simulink library "CTRL_SPECCTRL"  (R2024b)
settings: Solver=VariableStepAuto  StartTime=0.0  StopTime=10.0  RelTol=1e-3
libraries: CTRL_SPECCTRL_COND x1, CTRL_SPECCTRL_FB x1, CTRL_SPECCTRL_FF x1
settings Model: Creator=blatak  LastModifiedBy=blatak

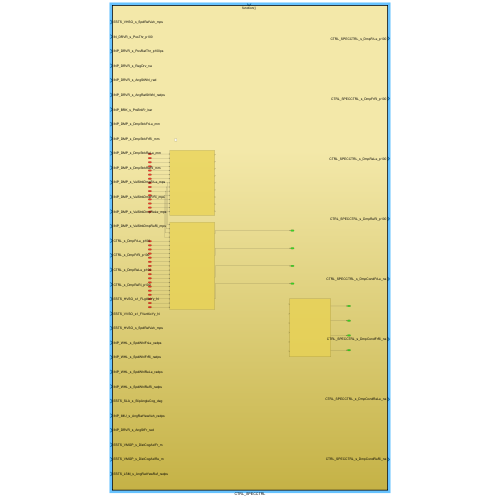
[thumbnail: Simulink's stored preview of the top-level diagram]
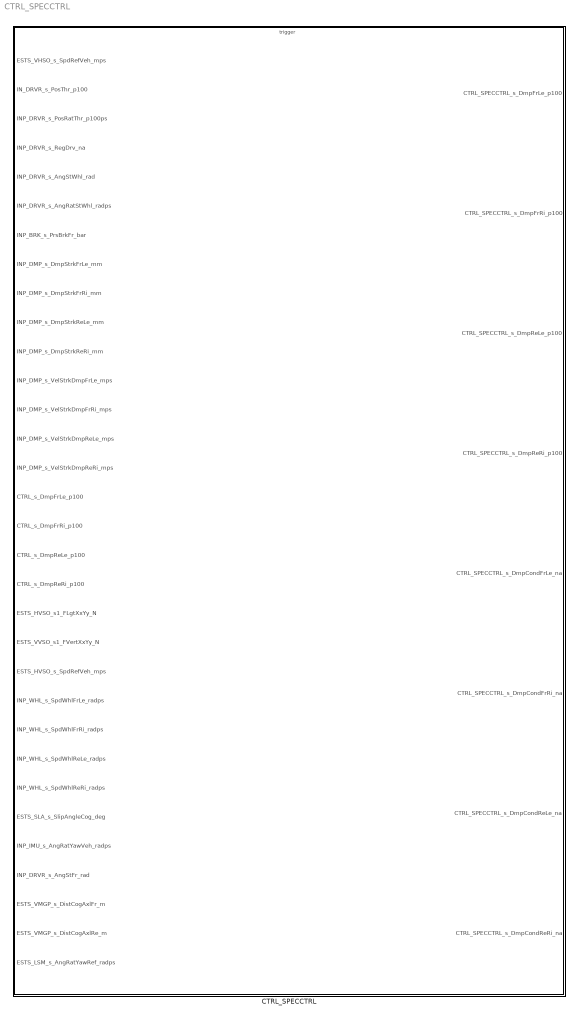
== system CTRL_SPECCTRL ==
  CTRL_SPECCTRL : Subsystem  TreatAsAtomicUnit=on

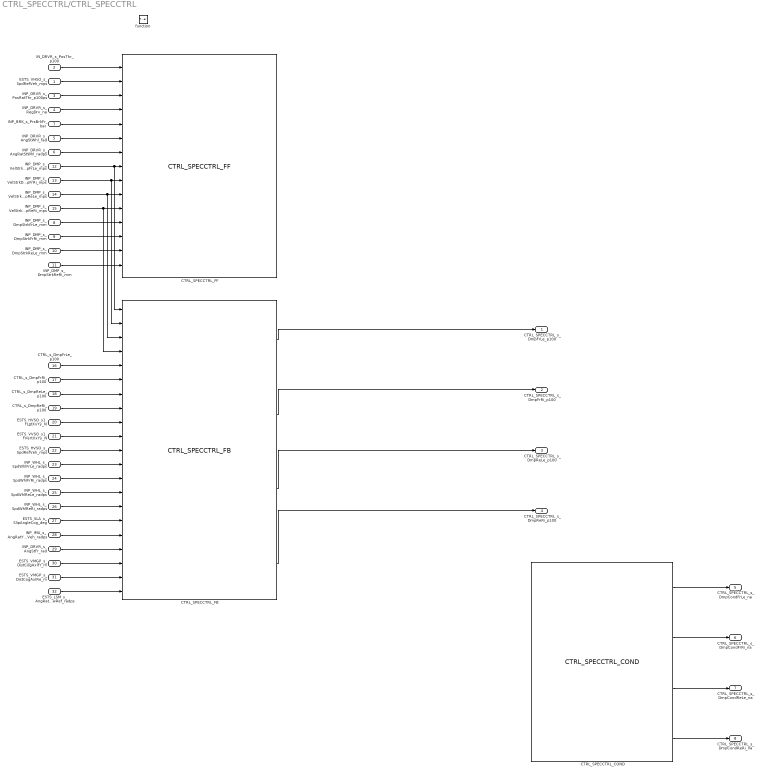
== system CTRL_SPECCTRL/CTRL_SPECCTRL ==
  ESTS_VHSO_s_SpdRefVeh_mps : Inport
  IN_DRVR_s_PosThr_p100 : Inport  Port=2
  INP_DRVR_s_PosRatThr_p100ps : Inport  Port=3
  INP_DRVR_s_RegDrv_na : Inport  Port=4
  INP_DRVR_s_AngStWhl_rad : Inport  Port=5
  INP_DRVR_s_AngRatStWhl_radps : Inport  Port=6
  INP_BRK_s_PrsBrkFr_bar : Inport  Port=7
  INP_DMP_s_DmpStrkFrLe_mm : Inport  Port=8
  INP_DMP_s_DmpStrkFrRi_mm : Inport  Port=9
  INP_DMP_s_DmpStrkReLe_mm : Inport  Port=10
  INP_DMP_s_DmpStrkReRi_mm : Inport  Port=11
  INP_DMP_s_VelStrkDmpFrLe_mps : Inport  Port=12
  INP_DMP_s_VelStrkDmpFrRi_mps : Inport  Port=13
  INP_DMP_s_VelStrkDmpReLe_mps : Inport  Port=14
  INP_DMP_s_VelStrkDmpReRi_mps : Inport  Port=15
  CTRL_s_DmpFrLe_p100 : Inport  Port=16
  CTRL_s_DmpFrRi_p100 : Inport  Port=17
  CTRL_s_DmpReLe_p100 : Inport  Port=18
  CTRL_s_DmpReRi_p100 : Inport  Port=19
  ESTS_HVSO_s1_FLgtXxYy_N : Inport  Port=20
  ESTS_VVSO_s1_FVertXxYy_N : Inport  Port=21
  ESTS_HVSO_s_SpdRefVeh_mps : Inport  Port=22
  INP_WHL_s_SpdWhlFrLe_radps : Inport  Port=23
  INP_WHL_s_SpdWhlFrRi_radps : Inport  Port=24
  INP_WHL_s_SpdWhlReLe_radps : Inport  Port=25
  INP_WHL_s_SpdWhlReRi_radps : Inport  Port=26
  ESTS_SLA_s_SlipAngleCog_deg : Inport  Port=27
  INP_IMU_s_AngRatYawVeh_radps : Inport  Port=28
  INP_DRVR_s_AngStFr_rad : Inport  Port=29
  ESTS_VMGP_s_DistCogAxlFr_m : Inport  Port=30
  ESTS_VMGP_s_DistCogAxlRe_m : Inport  Port=31
  ESTS_LSM_s_AngRatYawRef_radps : Inport  Port=32
  function : TriggerPort  TriggerType=function-call  VariantControl=(inherit)
  CTRL_SPECCTRL_COND : CTRL_SPECCTRL_COND/CTRL_SPECCTRL_COND  SystemSampleTime=-1  VariantActivationTime=update diagram  AllowFlexibleInterface=on  Latency=0  AutoFrameSizeCalculation=off
  CTRL_SPECCTRL_FB : CTRL_SPECCTRL_FB/CTRL_SPECCTRL_FB  SystemSampleTime=-1  VariantActivationTime=update diagram  AllowFlexibleInterface=on  Latency=0  AutoFrameSizeCalculation=off
  CTRL_SPECCTRL_FF : CTRL_SPECCTRL_FF/CTRL_SPECCTRL_FF  SystemSampleTime=-1  VariantActivationTime=update diagram  AllowFlexibleInterface=on  Latency=0  AutoFrameSizeCalculation=off
  CTRL_SPECCTRL_s_DmpFrLe_p100 : Outport
  CTRL_SPECCTRL_s_DmpFrRi_p100 : Outport  Port=2
  CTRL_SPECCTRL_s_DmpReLe_p100 : Outport  Port=3
  CTRL_SPECCTRL_s_DmpReRi_p100 : Outport  Port=4
  CTRL_SPECCTRL_s_DmpCondFrLe_na : Outport  Port=5
  CTRL_SPECCTRL_s_DmpCondFrRi_na : Outport  Port=6
  CTRL_SPECCTRL_s_DmpCondReLe_na : Outport  Port=7
  CTRL_SPECCTRL_s_DmpCondReRi_na : Outport  Port=8
  wires:
  CTRL_SPECCTRL_FB/1 -> CTRL_SPECCTRL_s_DmpFrLe_p100/1
  CTRL_SPECCTRL_FB/2 -> CTRL_SPECCTRL_s_DmpFrRi_p100/1
  CTRL_SPECCTRL_FB/3 -> CTRL_SPECCTRL_s_DmpReLe_p100/1
  CTRL_SPECCTRL_FB/4 -> CTRL_SPECCTRL_s_DmpReRi_p100/1
  IN_DRVR_s_PosThr_p100/1 -> CTRL_SPECCTRL_FF/1
  ESTS_VHSO_s_SpdRefVeh_mps/1 -> CTRL_SPECCTRL_FF/2
  INP_DRVR_s_PosRatThr_p100ps/1 -> CTRL_SPECCTRL_FF/3
  INP_DRVR_s_RegDrv_na/1 -> CTRL_SPECCTRL_FF/4
  INP_BRK_s_PrsBrkFr_bar/1 -> CTRL_SPECCTRL_FF/5
  INP_DRVR_s_AngStWhl_rad/1 -> CTRL_SPECCTRL_FF/6
  INP_DRVR_s_AngRatStWhl_radps/1 -> CTRL_SPECCTRL_FF/7
  INP_DMP_s_VelStrkDmpFrLe_mps/1 -> CTRL_SPECCTRL_FB/1, CTRL_SPECCTRL_FF/8
  INP_DMP_s_VelStrkDmpFrRi_mps/1 -> CTRL_SPECCTRL_FB/2, CTRL_SPECCTRL_FF/9
  INP_DMP_s_VelStrkDmpReLe_mps/1 -> CTRL_SPECCTRL_FB/3, CTRL_SPECCTRL_FF/10
  INP_DMP_s_VelStrkDmpReRi_mps/1 -> CTRL_SPECCTRL_FB/4, CTRL_SPECCTRL_FF/11
  INP_DMP_s_DmpStrkFrLe_mm/1 -> CTRL_SPECCTRL_FF/12
  INP_DMP_s_DmpStrkFrRi_mm/1 -> CTRL_SPECCTRL_FF/13
  INP_DMP_s_DmpStrkReLe_mm/1 -> CTRL_SPECCTRL_FF/14
  INP_DMP_s_DmpStrkReRi_mm/1 -> CTRL_SPECCTRL_FF/15
  CTRL_SPECCTRL_COND/1 -> CTRL_SPECCTRL_s_DmpCondFrLe_na/1
  CTRL_SPECCTRL_COND/2 -> CTRL_SPECCTRL_s_DmpCondFrRi_na/1
  CTRL_SPECCTRL_COND/3 -> CTRL_SPECCTRL_s_DmpCondReLe_na/1
  CTRL_SPECCTRL_COND/4 -> CTRL_SPECCTRL_s_DmpCondReRi_na/1
  CTRL_s_DmpFrLe_p100/1 -> CTRL_SPECCTRL_FB/5
  CTRL_s_DmpFrRi_p100/1 -> CTRL_SPECCTRL_FB/6
  CTRL_s_DmpReLe_p100/1 -> CTRL_SPECCTRL_FB/7
  CTRL_s_DmpReRi_p100/1 -> CTRL_SPECCTRL_FB/8
  ESTS_HVSO_s1_FLgtXxYy_N/1 -> CTRL_SPECCTRL_FB/9
  ESTS_VVSO_s1_FVertXxYy_N/1 -> CTRL_SPECCTRL_FB/10
  ESTS_HVSO_s_SpdRefVeh_mps/1 -> CTRL_SPECCTRL_FB/11
  INP_WHL_s_SpdWhlFrLe_radps/1 -> CTRL_SPECCTRL_FB/12
  INP_WHL_s_SpdWhlFrRi_radps/1 -> CTRL_SPECCTRL_FB/13
  INP_WHL_s_SpdWhlReLe_radps/1 -> CTRL_SPECCTRL_FB/14
  INP_WHL_s_SpdWhlReRi_radps/1 -> CTRL_SPECCTRL_FB/15
  ESTS_SLA_s_SlipAngleCog_deg/1 -> CTRL_SPECCTRL_FB/16
  INP_IMU_s_AngRatYawVeh_radps/1 -> CTRL_SPECCTRL_FB/17
  INP_DRVR_s_AngStFr_rad/1 -> CTRL_SPECCTRL_FB/18
  ESTS_VMGP_s_DistCogAxlFr_m/1 -> CTRL_SPECCTRL_FB/19
  ESTS_VMGP_s_DistCogAxlRe_m/1 -> CTRL_SPECCTRL_FB/20
  ESTS_LSM_s_AngRatYawRef_radps/1 -> CTRL_SPECCTRL_FB/21
